simulink library "motohawk_control_primitives_motoshare_lib"  (Simulink 6.3)
undefined symbols (not defined in the file or in its folder): motohawk_vardec_config_group, motohawk_vardec_path, p, samp_time, SampleTime
libraries: MotoHawk_lib x76, motohawk_control_primitives_lib x30, simulink x9
(part 1 of 3)
settings Model: Creator=Blake Suhre  LastModifiedBy=Jason_Tartt  StrictBusMsg=None

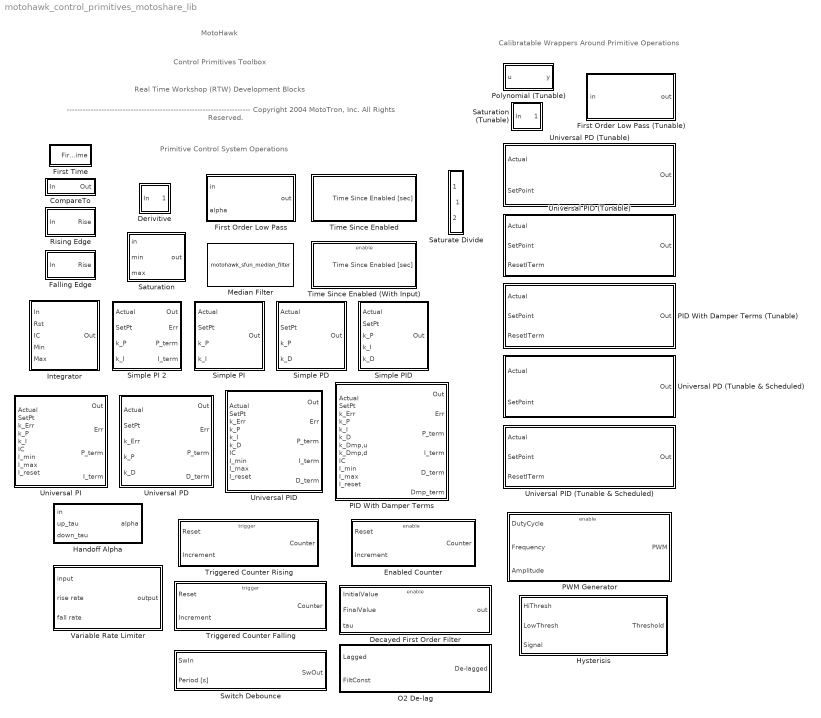
== system motohawk_control_primitives_motoshare_lib ==
  note: Calibratable Wrappers Around
      | Primitive Operations
  note: Primitive Control System Operations
  note: MotoHawk
  note: ---------------------------------------------------------------------
      | Copyright 2004 MotoTron, Inc.  All Rights Reserved.
  note: Real Time Workshop (RTW)
      | Development Blocks
  note: Control Primitives Toolbox
  CompareTo : Subsystem  mask(Equals){op===, val=1}
      mask prompts: op "Operator:"; val "Compare To:"
      mask help:
      | Check how input compares to 'n'.
      | Select an operation for comparison.
      | Any data type may be used for the value.  Real data type is based on input signal.
      mask init:
      | lbl = sprintf('in %s %d', op, double(val));
      | set_param([gcb '/RelOp'], 'Operator', op);
      mask StyleString: popup(==|~=|<|<=|>|>=),edit
      mask Display:
      | patch([0 0 1 1], 1.2*[0 0.075 0.075 0], [230/255 0/255 0/255])
      | patch([0 0 1 1], 1.2*[0.025 0.05 0.05 0.025], [150/255 0/255 0/255])
      | patch([0 0 1 1], 1.2*[0 0.025 0.025 0], [0/255 0/255 0/255])
      | 
      | disp(lbl);
  Decayed First Order Filter : Subsystem
      mask Type: Decayed First-Order Filter
      mask Description:
      | Discrete first-order low-pass filter that decays from the Initial Value to the Final Value when enabled.
      | 
      | The 'alpha' input is T/t.  So when alpha = 1, the block simply passes the input through to the output, and when alpha = 0, the block forever holds its last output value.
      mask Display:
      | patch([0 0 1 1], [0 0.075 0.075 0], [230/255 0/255 0/255])
      | patch([0 0 1 1], [0.025 0.05 0.05 0.025], [150/255 0/255 0/255])
      | patch([0 0 1 1], [0 0.025 0.025 0], [0/255 0/255 0/255])
      | 
      | disp('Decayed 1st-Order\nLow Pass');
  Derivitive : Subsystem  mask(Discrete Derivative){samp_time=SampleTime}
      mask prompts: samp_time "Sample Time"
      mask help:
      | Discrete-time derivitive.
      |
      | If 'Sample Time' is -1, then extra code and RAM will be generated to dynamically calculate dt.
      mask Display:
      | patch([0 0 1 1], [0 0.075 0.075 0], [230/255 0/255 0/255])
      | patch([0 0 1 1], [0.025 0.05 0.05 0.025], [150/255 0/255 0/255])
      | patch([0 0 1 1], [0 0.025 0.025 0], [0/255 0/255 0/255])
      | 
      | disp('\bf\itd/dt', 'texmode', 'on')
  Enabled Counter : Subsystem  TreatAsAtomicUnit=on
      mask Display:
      | patch([0 0 1 1], [0 0.075 0.075 0], [230/255 0/255 0/255])
      | patch([0 0 1 1], [0.025 0.05 0.05 0.025], [150/255 0/255 0/255])
      | patch([0 0 1 1], [0 0.025 0.025 0], [0/255 0/255 0/255])
      | 
      | disp(['ENABLED\nCOUNTER'])
  Falling Edge : Subsystem
      mask Display:
      | patch([0 0 1 1], [0 0.075 0.075 0], [230/255 0/255 0/255])
      | patch([0 0 1 1], [0.025 0.05 0.05 0.025], [150/255 0/255 0/255])
      | patch([0 0 1 1], [0 0.025 0.025 0], [0/255 0/255 0/255])
      | 
      | disp('Falling\nEdge');
  First Order Low Pass : Subsystem
      mask Type: First-Order Low-Pass Filter
      mask Description:
      | Discrete first-order low-pass filter.
      | 
      | The 'alpha' input is T/t.  So when alpha = 1, the block simply passes the input through to the output, and when alpha = 0, the block forever holds its last output value.
      mask Display:
      | patch([0 0 1 1], [0 0.075 0.075 0], [230/255 0/255 0/255])
      | patch([0 0 1 1], [0.025 0.05 0.05 0.025], [150/255 0/255 0/255])
      | patch([0 0 1 1], [0 0.025 0.025 0], [0/255 0/255 0/255])
      | 
      | disp('1st-Order\nLow Pass');
  First Order Low Pass (Tunable) : Subsystem  mask(First-Order Low-Pass Filter (Tunable)){nam='FiltConst', samp_time=-1, group=motohawk_vardec_path(gcb)}
      mask prompts: nam "Name"; samp_time "Sample Time"; group "MotoTune Group String"
      mask help:
      | Discrete first-order low-pass filter, with calibratable time-constant.
      |
      | If 'Sample Time' is -1, then extra code and RAM will be generated to dynamically calculate dt.
      mask Display:
      | patch([0 0 1 1], [0 0.075 0.075 0], [230/255 0/255 0/255])
      | patch([0 0 1 1], [0.025 0.05 0.05 0.025], [150/255 0/255 0/255])
      | patch([0 0 1 1], [0 0.025 0.025 0], [0/255 0/255 0/255])
      | 
      | disp('1st-Order\nLow Pass');
  First Time : Subsystem
      mask Display:
      | patch([0 0 1 1], [0 0.075 0.075 0], [230/255 0/255 0/255])
      | patch([0 0 1 1], [0.025 0.05 0.05 0.025], [150/255 0/255 0/255])
      | patch([0 0 1 1], [0 0.025 0.025 0], [0/255 0/255 0/255])
  Handoff Alpha : Subsystem  mask{samp_time=-1}
      mask prompts: samp_time "SampleTime"
      mask Display:
      | patch([0 0 1 1], [0 0.075 0.075 0], [230/255 0/255 0/255])
      | patch([0 0 1 1], [0.025 0.05 0.05 0.025], [150/255 0/255 0/255])
      | patch([0 0 1 1], [0 0.025 0.025 0], [0/255 0/255 0/255])
      | 
      | plot([.3 .4 .6 .8], [.3 .8 .8 .3]);
  Hysterisis : Subsystem
      mask Display:
      | patch([0 0 1 1], [0 0.075 0.075 0], [230/255 0/255 0/255])
      | patch([0 0 1 1], [0.025 0.05 0.05 0.025], [150/255 0/255 0/255])
      | patch([0 0 1 1], [0 0.025 0.025 0], [0/255 0/255 0/255])
      | 
      | disp('HYSTERISIS')
  Integrator : Subsystem  mask(Discrete Integrator){samp_time=samp_time}
      mask prompts: samp_time "Sample Time"
      mask help:
      | Resetable integrator with upper and lower windup limits.
      |
      | If 'Sample Time' is -1, then extra code and RAM will be generated to dynamically calculate dt.
      mask Display:
      | patch([0 0 1 1], 0.75*[0 0.075 0.075 0], [230/255 0/255 0/255])
      | patch([0 0 1 1], 0.75*[0.025 0.05 0.05 0.025], [150/255 0/255 0/255])
      | patch([0 0 1 1], 0.75*[0 0.025 0.025 0], [0/255 0/255 0/255])
      | 
      | disp('\fontsize{16}\bf\it\int dt', 'texmode', 'on')
  Median Filter : S-Function  FunctionName=motohawk_sfun_median_filter  Parameters=uint32(buffer_size)  mask(MotoHawk Median Filter){buffer_size=7}
      mask prompts: buffer_size "Buffer Size"
      mask help:
      | Maintains a buffer of 'Buffer Size' values, and outputs the median value stored in the buffer.
      |
      | ---------------------------------------------------------------------
      | Copyright 2004 MotoTron, Inc.  All Rights Reserved.
      mask init:
      | lbl = sprintf('Median Filter\nBuffer Size: %d', floor(double(buffer_size)));
      mask Display:
      | patch([0 0 1 1], [0 0.075 0.075 0], [230/255 0/255 0/255])
      | patch([0 0 1 1], [0.025 0.05 0.05 0.025], [150/255 0/255 0/255])
      | patch([0 0 1 1], [0 0.025 0.025 0], [0/255 0/255 0/255])
      | 
      | disp(lbl);
  O2 De-lag : Subsystem
      mask Display:
      | patch([0 0 1 1], [0 0.075 0.075 0], [230/255 0/255 0/255])
      | patch([0 0 1 1], [0.025 0.05 0.05 0.025], [150/255 0/255 0/255])
      | patch([0 0 1 1], [0 0.025 0.025 0], [0/255 0/255 0/255])
      | 
      | disp('First Order \nDe-Lag');
  PID With Damper Terms : Subsystem  Description=|  mask(PID with Damper Terms){samp_time=-1}
      | /* Name: ErrorGain Unit:mult ClassID:VAR StorageID:FLASH Access:RW4+RW3+NA2+NA1 TypeID:UINT4                   
      |    Gain:0.000000001 Min:0.000000000 Max:4.000000000 Format:10.9 UpdateID:REMOTE Help:"This gain is applied to "
      |    "the error term before it is used to calculate the P, I and D terms." VardecSig:6C */                       
      |                                                                                                                
      | /* Name: ITermLowerLim Unit:0 ClassID:VAR StorageID:FLASH Access:RW4+RW3+NA2+NA1 TypeID:SINT2 Gain:0.1         
      |    Min:-3276.8 Max:3276.7 Format:5.1 UpdateID:REMOTE Help:"Lower limit on the I-term value." VardecSig:6C */   
      |                                                                                                                
      | /* Name: ITermUpperLim ClassID:VAR StorageID:FLASH Access:RW4+RW3+NA2+NA1 TypeID:SINT2 Gain:0.1 Min:-3276.8    
      |    Max:3276.7 Format:5.1 UpdateID:REMOTE Help:"Upper limit on I-term value." VardecSig:6C */                   
      |                                                                                                                
      | /* Name: PIDOutLowerLim ClassID:VAR StorageID:FLASH Access:RW4+RW3+NA2+NA1 TypeID:SINT2 Gain:0.1               
      |    Min:-3276.8 Max:3276.7 Format:5.1 UpdateID:REMOTE Help:"Lower limit on PID output." VardecSig:6C */         
      |                                                                                                                
      | /* Name: PIDOutUpperLim ClassID:VAR StorageID:FLASH Access:RW4+RW3+NA2+NA1 TypeID:SINT2 Gain:0.1               
      |    Min:-3276.8 Max:3276.7 Format:3.1 UpdateID:REMOTE Help:"Upper limit on PID output." VardecSig:6C */         
      |                                                                                                                
      | /* Name: PIDError ClassID:VAR StorageID:RAM Access:RO4+RO3+NA2+NA1 TypeID:SINT2 Gain:1 Min:-32768.00           
      |    Max:32767.00 Format:4.2 UpdateID:BACKGND Help:"Current controller error input value." VardecSig:6C */       
      |                                                                                                                
      | /* Name: PTerm ClassID:VAR StorageID:RAM Access:RO4+RO3+NA2+NA1 TypeID:SINT2 Gain:1 Min:-32768.00              
      |    Max:32767.00 Format:4.2 UpdateID:BACKGND Help:"Current P-term value" VardecSig:6C */                        
      |                                                                                                                
      | /* Name: ITerm ClassID:VAR StorageID:RAM Access:RO4+RO3+NA2+NA1 TypeID:SINT2 Gain:1 Min:-32768.00              
      |    Max:32767.00 Format:4.2 UpdateID:BACKGND Help:"Current I-term value" VardecSig:6C */                        
      |                                                                                                                
      | /* Name: DTerm ClassID:VAR StorageID:RAM Access:RO4+RO3+NA2+NA1 TypeID:SINT2 Gain:1 Min:-32768.00              
      |    Max:32767.00 Format:4.2 UpdateID:BACKGND Help:"Current D-term value" VardecSig:6C */                        
      |                                                                                                                
      | /* Name: DamperTerm ClassID:VAR StorageID:RAM Access:RO4+RO3+NA2+NA1 TypeID:SINT2 Gain:1 Min:-32768.00         
      |    Max:32767.00 Format:4.2 UpdateID:BACKGND Help:"Current Damper-term value" VardecSig:6C */                   
      |                                                                                                                
      | /* Name: PIDOutput ClassID:VAR StorageID:FLASH Access:RW4+RW3+NA2+NA1 TypeID:SINT2 Gain:1 Min:-32768.00        
      |    Max:32767.00 Format:4.2 UpdateID:REMOTE Help:"PID current output." VardecSig:6C */
      mask prompts: samp_time "Sample Time"
      mask help:
      | Resettable PID controller with damper terms and limits on the I-term.
      |
      | If 'Sample Time' is -1, then extra code and RAM will be generated to dynamically calculate dt.
      mask Display:
      | patch([0 0 1 1], 0.5*[0 0.075 0.075 0], [230/255 0/255 0/255])
      | patch([0 0 1 1], 0.5*[0.025 0.05 0.05 0.025], [150/255 0/255 0/255])
      | patch([0 0 1 1], 0.5*[0 0.025 0.025 0], [0/255 0/255 0/255])
      | 
      | disp('\fontsize{16}\bf\itPIDD', 'texmode', 'on')
  PID With Damper Terms (Tunable) : Subsystem  mask(PID with Damper Terms (Tunable)){nam='Electronic Throttle Control', prefix='ETC_', samp_time=-1, units='', grp='Actuators | ETC'}
      mask prompts: nam "Name"; samp_time "Sample Time"; grp "MotoTune Group String"
      mask help:
      | This block wraps a 'PID With Damper Terms' block to provide calibrations and probes for most parameters.
      |
      | If 'Sample Time' is -1, then extra code and RAM will be generated to dynamically calculate dt.
      mask Display:
      | patch([0 0 1 1], [0 0.075 0.075 0], [230/255 0/255 0/255])
      | patch([0 0 1 1], [0.025 0.05 0.05 0.025], [150/255 0/255 0/255])
      | patch([0 0 1 1], [0 0.025 0.025 0], [0/255 0/255 0/255])
      | 
      | disp([nam '\n(PIDD)']);
  PWM Generator : Subsystem  TreatAsAtomicUnit=on
      mask Display:
      | patch([0 0 1 1], [0 0.075 0.075 0], [230/255 0/255 0/255])
      | patch([0 0 1 1], [0.025 0.05 0.05 0.025], [150/255 0/255 0/255])
      | patch([0 0 1 1], [0 0.025 0.025 0], [0/255 0/255 0/255])
      | 
      | disp('ENABLED\nPWM\nGENERATOR')
  Polynomial (Tunable) : Subsystem  mask(Polynomial (Tunable)){prefix='SamplePoly', numcoef=6, grp=motohawk_vardec_path(gcb)}
      mask prompts: numcoef "Number Of Coefficients"; grp "MotoTune Group String"
      mask help: Polynomial evaluation block with calibratable coefficients and centering/scaling parameters.
      mask Display:
      | patch([0 0 1 1], [0 0.075 0.075 0], [230/255 0/255 0/255])
      | patch([0 0 1 1], [0.025 0.05 0.05 0.025], [150/255 0/255 0/255])
      | patch([0 0 1 1], [0 0.025 0.025 0], [0/255 0/255 0/255])
      | 
      | disp(['P(u)\nO(P)'])
  Rising Edge : Subsystem
      mask Display:
      | patch([0 0 1 1], [0 0.075 0.075 0], [230/255 0/255 0/255])
      | patch([0 0 1 1], [0.025 0.05 0.05 0.025], [150/255 0/255 0/255])
      | patch([0 0 1 1], [0 0.025 0.025 0], [0/255 0/255 0/255])
      | 
      | disp('Rising\nEdge');
  Saturate Divide : Subsystem
      mask Display:
      | patch([0 0 1 1], [0 0.075 0.075 0], [230/255 0/255 0/255])
      | patch([0 0 1 1], [0.025 0.05 0.05 0.025], [150/255 0/255 0/255])
      | patch([0 0 1 1], [0 0.025 0.025 0], [0/255 0/255 0/255])
  Saturation : Subsystem  mask(Saturation){}
      mask help: Saturation block.
      mask Display:
      | patch([0 0 1 1], [0 0.075 0.075 0], [230/255 0/255 0/255])
      | patch([0 0 1 1], [0.025 0.05 0.05 0.025], [150/255 0/255 0/255])
      | patch([0 0 1 1], [0 0.025 0.025 0], [0/255 0/255 0/255])
      | 
      | plot([.2 .4 .6 .8], [.2 .2 .9 .9])
  Saturation (Tunable) : Subsystem  mask(Saturation (Tunable)){prefix='Saturation', units='', grp=motohawk_vardec_path(gcb)}
      mask prompts: grp "MotoTune Group String"
      mask help: Saturation block with calibratable min/max values.
      mask Display:
      | patch([0 0 1 1], [0 0.075 0.075 0], [230/255 0/255 0/255])
      | patch([0 0 1 1], [0.025 0.05 0.05 0.025], [150/255 0/255 0/255])
      | patch([0 0 1 1], [0 0.025 0.025 0], [0/255 0/255 0/255])
      | 
      | plot([0 .2 .8 1], [.1 .1 1 1])
  Simple PD : Subsystem  Description=|  mask(Universal PD){samp_time=-1}
      | /* Name: ErrorGain Unit:mult ClassID:VAR StorageID:FLASH Access:RW4+RW3+NA2+NA1 TypeID:UINT4                   
      |    Gain:0.000000001 Min:0.000000000 Max:4.000000000 Format:10.9 UpdateID:REMOTE Help:"This gain is applied to "
      |    "the error term before it is used to calculate the P, I and D terms." VardecSig:6C */                       
      |                                                                                                                
      | /* Name: ITermLowerLim Unit:0 ClassID:VAR StorageID:FLASH Access:RW4+RW3+NA2+NA1 TypeID:SINT2 Gain:0.1         
      |    Min:-3276.8 Max:3276.7 Format:5.1 UpdateID:REMOTE Help:"Lower limit on the I-term value." VardecSig:6C */   
      |                                                                                                                
      | /* Name: ITermUpperLim ClassID:VAR StorageID:FLASH Access:RW4+RW3+NA2+NA1 TypeID:SINT2 Gain:0.1 Min:-3276.8    
      |    Max:3276.7 Format:5.1 UpdateID:REMOTE Help:"Upper limit on I-term value." VardecSig:6C */                   
      |                                                                                                                
      | /* Name: PIDOutLowerLim ClassID:VAR StorageID:FLASH Access:RW4+RW3+NA2+NA1 TypeID:SINT2 Gain:0.1               
      |    Min:-3276.8 Max:3276.7 Format:5.1 UpdateID:REMOTE Help:"Lower limit on PID output." VardecSig:6C */         
      |                                                                                                                
      | /* Name: PIDOutUpperLim ClassID:VAR StorageID:FLASH Access:RW4+RW3+NA2+NA1 TypeID:SINT2 Gain:0.1               
      |    Min:-3276.8 Max:3276.7 Format:3.1 UpdateID:REMOTE Help:"Upper limit on PID output." VardecSig:6C */
      mask prompts: samp_time "Sample Time"
      mask help:
      | Resettable PD controller.
      |
      | If 'Sample Time' is -1, then extra code and RAM will be generated to dynamically calculate dt.
      mask Display:
      | patch([0 0 1 1], 0.75*[0 0.075 0.075 0], [230/255 0/255 0/255])
      | patch([0 0 1 1], 0.75*[0.025 0.05 0.05 0.025], [150/255 0/255 0/255])
      | patch([0 0 1 1], 0.75*[0 0.025 0.025 0], [0/255 0/255 0/255])
      | 
      | disp('\fontsize{16}\bf\itPD', 'texmode', 'on');
  Simple PI : Subsystem  Description=|  mask(Universal PID){samp_time=-1}
      | /* Name: ErrorGain Unit:mult ClassID:VAR StorageID:FLASH Access:RW4+RW3+NA2+NA1 TypeID:UINT4                   
      |    Gain:0.000000001 Min:0.000000000 Max:4.000000000 Format:10.9 UpdateID:REMOTE Help:"This gain is applied to "
      |    "the error term before it is used to calculate the P, I and D terms." VardecSig:6C */                       
      |                                                                                                                
      | /* Name: ITermLowerLim Unit:0 ClassID:VAR StorageID:FLASH Access:RW4+RW3+NA2+NA1 TypeID:SINT2 Gain:0.1         
      |    Min:-3276.8 Max:3276.7 Format:5.1 UpdateID:REMOTE Help:"Lower limit on the I-term value." VardecSig:6C */   
      |                                                                                                                
      | /* Name: ITermUpperLim ClassID:VAR StorageID:FLASH Access:RW4+RW3+NA2+NA1 TypeID:SINT2 Gain:0.1 Min:-3276.8    
      |    Max:3276.7 Format:5.1 UpdateID:REMOTE Help:"Upper limit on I-term value." VardecSig:6C */                   
      |                                                                                                                
      | /* Name: PIDOutLowerLim ClassID:VAR StorageID:FLASH Access:RW4+RW3+NA2+NA1 TypeID:SINT2 Gain:0.1               
      |    Min:-3276.8 Max:3276.7 Format:5.1 UpdateID:REMOTE Help:"Lower limit on PID output." VardecSig:6C */         
      |                                                                                                                
      | /* Name: PIDOutUpperLim ClassID:VAR StorageID:FLASH Access:RW4+RW3+NA2+NA1 TypeID:SINT2 Gain:0.1               
      |    Min:-3276.8 Max:3276.7 Format:3.1 UpdateID:REMOTE Help:"Upper limit on PID output." VardecSig:6C */
      mask prompts: samp_time "Sample Time"
      mask help:
      | Resettable PID controller with limits on the I-term.
      |
      | If 'Sample Time' is -1, then extra code and RAM will be generated to dynamically calculate dt.
      mask Display:
      | patch([0 0 1 1], 0.75*[0 0.075 0.075 0], [230/255 0/255 0/255])
      | patch([0 0 1 1], 0.75*[0.025 0.05 0.05 0.025], [150/255 0/255 0/255])
      | patch([0 0 1 1], 0.75*[0 0.025 0.025 0], [0/255 0/255 0/255])
      | 
      | disp('\fontsize{16}\bf\itPI', 'texmode', 'on');
  Simple PI 2 : Subsystem  Description=|  mask(Universal PID){samp_time=-1}
      | /* Name: ErrorGain Unit:mult ClassID:VAR StorageID:FLASH Access:RW4+RW3+NA2+NA1 TypeID:UINT4                   
      |    Gain:0.000000001 Min:0.000000000 Max:4.000000000 Format:10.9 UpdateID:REMOTE Help:"This gain is applied to "
      |    "the error term before it is used to calculate the P, I and D terms." VardecSig:6C */                       
      |                                                                                                                
      | /* Name: ITermLowerLim Unit:0 ClassID:VAR StorageID:FLASH Access:RW4+RW3+NA2+NA1 TypeID:SINT2 Gain:0.1         
      |    Min:-3276.8 Max:3276.7 Format:5.1 UpdateID:REMOTE Help:"Lower limit on the I-term value." VardecSig:6C */   
      |                                                                                                                
      | /* Name: ITermUpperLim ClassID:VAR StorageID:FLASH Access:RW4+RW3+NA2+NA1 TypeID:SINT2 Gain:0.1 Min:-3276.8    
      |    Max:3276.7 Format:5.1 UpdateID:REMOTE Help:"Upper limit on I-term value." VardecSig:6C */                   
      |                                                                                                                
      | /* Name: PIDOutLowerLim ClassID:VAR StorageID:FLASH Access:RW4+RW3+NA2+NA1 TypeID:SINT2 Gain:0.1               
      |    Min:-3276.8 Max:3276.7 Format:5.1 UpdateID:REMOTE Help:"Lower limit on PID output." VardecSig:6C */         
      |                                                                                                                
      | /* Name: PIDOutUpperLim ClassID:VAR StorageID:FLASH Access:RW4+RW3+NA2+NA1 TypeID:SINT2 Gain:0.1               
      |    Min:-3276.8 Max:3276.7 Format:3.1 UpdateID:REMOTE Help:"Upper limit on PID output." VardecSig:6C */
      mask prompts: samp_time "Sample Time"
      mask help:
      | Resettable PID controller with limits on the I-term.
      |
      | If 'Sample Time' is -1, then extra code and RAM will be generated to dynamically calculate dt.
      mask Display:
      | patch([0 0 1 1], 0.75*[0 0.075 0.075 0], [230/255 0/255 0/255])
      | patch([0 0 1 1], 0.75*[0.025 0.05 0.05 0.025], [150/255 0/255 0/255])
      | patch([0 0 1 1], 0.75*[0 0.025 0.025 0], [0/255 0/255 0/255])
      | 
      | disp('\fontsize{16}\bf\itPI', 'texmode', 'on');
  Simple PID : Subsystem  Description=|  mask(Universal PID){samp_time=-1}
      | /* Name: ErrorGain Unit:mult ClassID:VAR StorageID:FLASH Access:RW4+RW3+NA2+NA1 TypeID:UINT4                   
      |    Gain:0.000000001 Min:0.000000000 Max:4.000000000 Format:10.9 UpdateID:REMOTE Help:"This gain is applied to "
      |    "the error term before it is used to calculate the P, I and D terms." VardecSig:6C */                       
      |                                                                                                                
      | /* Name: ITermLowerLim Unit:0 ClassID:VAR StorageID:FLASH Access:RW4+RW3+NA2+NA1 TypeID:SINT2 Gain:0.1         
      |    Min:-3276.8 Max:3276.7 Format:5.1 UpdateID:REMOTE Help:"Lower limit on the I-term value." VardecSig:6C */   
      |                                                                                                                
      | /* Name: ITermUpperLim ClassID:VAR StorageID:FLASH Access:RW4+RW3+NA2+NA1 TypeID:SINT2 Gain:0.1 Min:-3276.8    
      |    Max:3276.7 Format:5.1 UpdateID:REMOTE Help:"Upper limit on I-term value." VardecSig:6C */                   
      |                                                                                                                
      | /* Name: PIDOutLowerLim ClassID:VAR StorageID:FLASH Access:RW4+RW3+NA2+NA1 TypeID:SINT2 Gain:0.1               
      |    Min:-3276.8 Max:3276.7 Format:5.1 UpdateID:REMOTE Help:"Lower limit on PID output." VardecSig:6C */         
      |                                                                                                                
      | /* Name: PIDOutUpperLim ClassID:VAR StorageID:FLASH Access:RW4+RW3+NA2+NA1 TypeID:SINT2 Gain:0.1               
      |    Min:-3276.8 Max:3276.7 Format:3.1 UpdateID:REMOTE Help:"Upper limit on PID output." VardecSig:6C */
      mask prompts: samp_time "Sample Time"
      mask help:
      | Resettable PID controller with limits on the I-term.
      |
      | If 'Sample Time' is -1, then extra code and RAM will be generated to dynamically calculate dt.
      mask Display:
      | patch([0 0 1 1], 0.75*[0 0.075 0.075 0], [230/255 0/255 0/255])
      | patch([0 0 1 1], 0.75*[0.025 0.05 0.05 0.025], [150/255 0/255 0/255])
      | patch([0 0 1 1], 0.75*[0 0.025 0.025 0], [0/255 0/255 0/255])
      | 
      | disp('\fontsize{16}\bf\itPID', 'texmode', 'on');
  Switch Debounce : Subsystem
      mask Display:
      | patch([0 0 1 1], [0 0.075 0.075 0], [230/255 0/255 0/255])
      | patch([0 0 1 1], [0.025 0.05 0.05 0.025], [150/255 0/255 0/255])
      | patch([0 0 1 1], [0 0.025 0.025 0], [0/255 0/255 0/255])
      | 
      | disp('SWITCH DEBOUNCE');
  Time Since Enabled : Subsystem  mask(Time Since Enabled){samp_time=-1}
      mask prompts: samp_time "Sample Time"
      mask help:
      | Outputs the amount of time that has elapsed since the enable input has gone high.
      |
      | Holds its value when the enable input goes low, but resets again when it goes high.
      |
      | If 'Sample Time' is -1, then extra code and RAM will be generated to dynamically calculate dt.
      mask Display:
      | patch([0 0 1 1], [0 0.075 0.075 0], [230/255 0/255 0/255])
      | patch([0 0 1 1], [0.025 0.05 0.05 0.025], [150/255 0/255 0/255])
      | patch([0 0 1 1], [0 0.025 0.025 0], [0/255 0/255 0/255])
      | 
      | disp('Time Since Enabled\n[sec]');
  Time Since Enabled (With Input) : Subsystem  mask(Time Since Enabled){samp_time=-1, init=0}
      mask prompts: samp_time "Sample Time"; init "Output When Disabled"
      mask help:
      | Outputs the amount of time that has elapsed since the enable input has gone high.
      |
      | Holds its value when the enable input goes low, but resets again when it goes high.
      |
      | If 'Sample Time' is -1, then extra code and RAM will be generated to dynamically calculate dt.
      mask Display:
      | patch([0 0 1 1], [0 0.075 0.075 0], [230/255 0/255 0/255])
      | patch([0 0 1 1], [0.025 0.05 0.05 0.025], [150/255 0/255 0/255])
      | patch([0 0 1 1], [0 0.025 0.025 0], [0/255 0/255 0/255])
      | 
      | disp('Time Since Enabled\n[sec]');
  Triggered Counter Falling : Subsystem  TreatAsAtomicUnit=on
      mask Type: MotoHawk Engine Physics:  No Adapt Counter
      mask Description:
      | ---------------------------------------------------------------------
      | Copyright 2004 MotoTron Corp.  All Rights Reserved.
      mask Display:
      | patch([0 0 1 1], [0 0.075 0.075 0], [230/255 0/255 0/255])
      | patch([0 0 1 1], [0.025 0.05 0.05 0.025], [150/255 0/255 0/255])
      | patch([0 0 1 1], [0 0.025 0.025 0], [0/255 0/255 0/255])
      | 
      | disp(['TRIGGERED\nCOUNTER\n(Falling Edge)'])
  Triggered Counter Rising : Subsystem  TreatAsAtomicUnit=on
      mask Type: MotoHawk Engine Physics:  No Adapt Counter
      mask Description:
      | ---------------------------------------------------------------------
      | Copyright 2004 MotoTron Corp.  All Rights Reserved.
      mask Display:
      | patch([0 0 1 1], [0 0.075 0.075 0], [230/255 0/255 0/255])
      | patch([0 0 1 1], [0.025 0.05 0.05 0.025], [150/255 0/255 0/255])
      | patch([0 0 1 1], [0 0.025 0.025 0], [0/255 0/255 0/255])
      | 
      | disp(['TRIGGERED\nCOUNTER\n(Rising Edge)'])
  Universal PD : Subsystem  Description=|  mask(Universal PD){samp_time=-1}
      | /* Name: ErrorGain Unit:mult ClassID:VAR StorageID:FLASH Access:RW4+RW3+NA2+NA1 TypeID:UINT4                   
      |    Gain:0.000000001 Min:0.000000000 Max:4.000000000 Format:10.9 UpdateID:REMOTE Help:"This gain is applied to "
      |    "the error term before it is used to calculate the P, I and D terms." VardecSig:6C */                       
      |                                                                                                                
      | /* Name: ITermLowerLim Unit:0 ClassID:VAR StorageID:FLASH Access:RW4+RW3+NA2+NA1 TypeID:SINT2 Gain:0.1         
      |    Min:-3276.8 Max:3276.7 Format:5.1 UpdateID:REMOTE Help:"Lower limit on the I-term value." VardecSig:6C */   
      |                                                                                                                
      | /* Name: ITermUpperLim ClassID:VAR StorageID:FLASH Access:RW4+RW3+NA2+NA1 TypeID:SINT2 Gain:0.1 Min:-3276.8    
      |    Max:3276.7 Format:5.1 UpdateID:REMOTE Help:"Upper limit on I-term value." VardecSig:6C */                   
      |                                                                                                                
      | /* Name: PIDOutLowerLim ClassID:VAR StorageID:FLASH Access:RW4+RW3+NA2+NA1 TypeID:SINT2 Gain:0.1               
      |    Min:-3276.8 Max:3276.7 Format:5.1 UpdateID:REMOTE Help:"Lower limit on PID output." VardecSig:6C */         
      |                                                                                                                
      | /* Name: PIDOutUpperLim ClassID:VAR StorageID:FLASH Access:RW4+RW3+NA2+NA1 TypeID:SINT2 Gain:0.1               
      |    Min:-3276.8 Max:3276.7 Format:3.1 UpdateID:REMOTE Help:"Upper limit on PID output." VardecSig:6C */
      mask prompts: samp_time "Sample Time"
      mask help:
      | Resettable PD controller.
      |
      | If 'Sample Time' is -1, then extra code and RAM will be generated to dynamically calculate dt.
      mask Display:
      | patch([0 0 1 1], 0.5*[0 0.075 0.075 0], [230/255 0/255 0/255])
      | patch([0 0 1 1], 0.5*[0.025 0.05 0.05 0.025], [150/255 0/255 0/255])
      | patch([0 0 1 1], 0.5*[0 0.025 0.025 0], [0/255 0/255 0/255])
      | 
      | disp('\fontsize{16}\bf\itPD', 'texmode', 'on');
  Universal PD (Tunable & Scheduled) : Subsystem  mask(Universal PD (Tunable)){nam='Idle Spark PD', prefix='IdleSpark_', samp_time=SampleTime, units='degCA', tblsize=10, group='Engine Control | Run | Idle Control'}
      mask prompts: nam "Name"; samp_time "Sample Time"; tblsize "Gain Schedule Table Size"; group "MotoTune Group String"
      mask help:
      | This block wraps a 'Universal PD' block to provide gain scheduling and calibrations and probes for most parameters.
      |
      | If 'Sample Time' is -1, then extra code and RAM will be generated to dynamically calculate dt.
      mask init:
      | grp = [group ' | ' nam];
      mask Display:
      | patch([0 0 1 1], [0 0.075 0.075 0], [230/255 0/255 0/255])
      | patch([0 0 1 1], [0.025 0.05 0.05 0.025], [150/255 0/255 0/255])
      | patch([0 0 1 1], [0 0.025 0.025 0], [0/255 0/255 0/255])
      | 
      | disp([nam '\n(PD w/ Gain Schedules)']);
  Universal PD (Tunable) : Subsystem  mask(Universal PD (Tunable)){nam='Idle Spark Control', prefix='IdleSpark_', samp_time=SampleTime, units='', group='Engine Control | Run | Idle Control'}
      mask prompts: nam "Name"; samp_time "Sample Time"; group "MotoTune Group String"
      mask help:
      | This block wraps a 'Universal PD' block to provide calibrations and probes for most parameters.
      |
      | If 'Sample Time' is -1, then extra code and RAM will be generated to dynamically calculate dt.
      mask init:
      | grp = [group ' | ' nam];
      mask Display:
      | patch([0 0 1 1], [0 0.075 0.075 0], [230/255 0/255 0/255])
      | patch([0 0 1 1], [0.025 0.05 0.05 0.025], [150/255 0/255 0/255])
      | patch([0 0 1 1], [0 0.025 0.025 0], [0/255 0/255 0/255])
      | 
      | disp([nam '\n(PD)']);
  Universal PI : Subsystem  Description=|  mask(Universal PID){samp_time=-1}
      | /* Name: ErrorGain Unit:mult ClassID:VAR StorageID:FLASH Access:RW4+RW3+NA2+NA1 TypeID:UINT4                   
      |    Gain:0.000000001 Min:0.000000000 Max:4.000000000 Format:10.9 UpdateID:REMOTE Help:"This gain is applied to "
      |    "the error term before it is used to calculate the P, I and D terms." VardecSig:6C */                       
      |                                                                                                                
      | /* Name: ITermLowerLim Unit:0 ClassID:VAR StorageID:FLASH Access:RW4+RW3+NA2+NA1 TypeID:SINT2 Gain:0.1         
      |    Min:-3276.8 Max:3276.7 Format:5.1 UpdateID:REMOTE Help:"Lower limit on the I-term value." VardecSig:6C */   
      |                                                                                                                
      | /* Name: ITermUpperLim ClassID:VAR StorageID:FLASH Access:RW4+RW3+NA2+NA1 TypeID:SINT2 Gain:0.1 Min:-3276.8    
      |    Max:3276.7 Format:5.1 UpdateID:REMOTE Help:"Upper limit on I-term value." VardecSig:6C */                   
      |                                                                                                                
      | /* Name: PIDOutLowerLim ClassID:VAR StorageID:FLASH Access:RW4+RW3+NA2+NA1 TypeID:SINT2 Gain:0.1               
      |    Min:-3276.8 Max:3276.7 Format:5.1 UpdateID:REMOTE Help:"Lower limit on PID output." VardecSig:6C */         
      |                                                                                                                
      | /* Name: PIDOutUpperLim ClassID:VAR StorageID:FLASH Access:RW4+RW3+NA2+NA1 TypeID:SINT2 Gain:0.1               
      |    Min:-3276.8 Max:3276.7 Format:3.1 UpdateID:REMOTE Help:"Upper limit on PID output." VardecSig:6C */
      mask prompts: samp_time "Sample Time"
      mask help:
      | Resettable PID controller with limits on the I-term.
      |
      | If 'Sample Time' is -1, then extra code and RAM will be generated to dynamically calculate dt.
      mask Display:
      | patch([0 0 1 1], 0.5*[0 0.075 0.075 0], [230/255 0/255 0/255])
      | patch([0 0 1 1], 0.5*[0.025 0.05 0.05 0.025], [150/255 0/255 0/255])
      | patch([0 0 1 1], 0.5*[0 0.025 0.025 0], [0/255 0/255 0/255])
      | 
      | disp('\fontsize{16}\bf\itPI', 'texmode', 'on');
  Universal PID : Subsystem  Description=|  mask(Universal PID){samp_time=-1}
      | /* Name: ErrorGain Unit:mult ClassID:VAR StorageID:FLASH Access:RW4+RW3+NA2+NA1 TypeID:UINT4                   
      |    Gain:0.000000001 Min:0.000000000 Max:4.000000000 Format:10.9 UpdateID:REMOTE Help:"This gain is applied to "
      |    "the error term before it is used to calculate the P, I and D terms." VardecSig:6C */                       
      |                                                                                                                
      | /* Name: ITermLowerLim Unit:0 ClassID:VAR StorageID:FLASH Access:RW4+RW3+NA2+NA1 TypeID:SINT2 Gain:0.1         
      |    Min:-3276.8 Max:3276.7 Format:5.1 UpdateID:REMOTE Help:"Lower limit on the I-term value." VardecSig:6C */   
      |                                                                                                                
      | /* Name: ITermUpperLim ClassID:VAR StorageID:FLASH Access:RW4+RW3+NA2+NA1 TypeID:SINT2 Gain:0.1 Min:-3276.8    
      |    Max:3276.7 Format:5.1 UpdateID:REMOTE Help:"Upper limit on I-term value." VardecSig:6C */                   
      |                                                                                                                
      | /* Name: PIDOutLowerLim ClassID:VAR StorageID:FLASH Access:RW4+RW3+NA2+NA1 TypeID:SINT2 Gain:0.1               
      |    Min:-3276.8 Max:3276.7 Format:5.1 UpdateID:REMOTE Help:"Lower limit on PID output." VardecSig:6C */         
      |                                                                                                                
      | /* Name: PIDOutUpperLim ClassID:VAR StorageID:FLASH Access:RW4+RW3+NA2+NA1 TypeID:SINT2 Gain:0.1               
      |    Min:-3276.8 Max:3276.7 Format:3.1 UpdateID:REMOTE Help:"Upper limit on PID output." VardecSig:6C */
      mask prompts: samp_time "Sample Time"
      mask help:
      | Resettable PID controller with limits on the I-term.
      |
      | If 'Sample Time' is -1, then extra code and RAM will be generated to dynamically calculate dt.
      mask Display:
      | patch([0 0 1 1], 0.5*[0 0.075 0.075 0], [230/255 0/255 0/255])
      | patch([0 0 1 1], 0.5*[0.025 0.05 0.05 0.025], [150/255 0/255 0/255])
      | patch([0 0 1 1], 0.5*[0 0.025 0.025 0], [0/255 0/255 0/255])
      | 
      | disp('\fontsize{16}\bf\itPID', 'texmode', 'on');
  Universal PID (Tunable & Scheduled) : Subsystem  mask(Universal PID (Tunable)){nam='Idle Air PID', prefix='IdleAir_', samp_time=SampleTime, units='%', tblsize=10, group='Engine Control | Run | Idle Control'}
      mask prompts: nam "Name"; samp_time "Sample Time"; tblsize "Gain Schedule Table Size"; group "MotoTune Group String"
      mask help:
      | This block wraps a 'Universal PID' block to provide gain scheduling and calibrations and probes for most parameters.
      |
      | If 'Sample Time' is -1, then extra code and RAM will be generated to dynamically calculate dt.
      mask init:
      | grp = [group ' | ' nam];
      mask Display:
      | patch([0 0 1 1], [0 0.075 0.075 0], [230/255 0/255 0/255])
      | patch([0 0 1 1], [0.025 0.05 0.05 0.025], [150/255 0/255 0/255])
      | patch([0 0 1 1], [0 0.025 0.025 0], [0/255 0/255 0/255])
      | 
      | disp([nam '\n(PID w/ Gain Schedules)']);
  Universal PID (Tunable) : Subsystem  mask(Universal PID (Tunable)){nam='Idle Air Control', prefix='IdleAir_', samp_time=SampleTime, units='', group='Engine Control | Run | Idle Control'}
      mask prompts: nam "Name"; samp_time "Sample Time"; group "MotoTune Group String"
      mask help:
      | This block wraps a 'Universal PID' block to provide calibrations and probes for most parameters.
      |
      | If 'Sample Time' is -1, then extra code and RAM will be generated to dynamically calculate dt.
      mask init:
      | grp = [group ' | ' nam];
      mask Display:
      | patch([0 0 1 1], [0 0.075 0.075 0], [230/255 0/255 0/255])
      | patch([0 0 1 1], [0.025 0.05 0.05 0.025], [150/255 0/255 0/255])
      | patch([0 0 1 1], [0 0.025 0.025 0], [0/255 0/255 0/255])
      | 
      | disp([nam '\n(PID)']);
  Variable Rate Limiter : Subsystem  mask(Variable Rate Limiter){}
      mask help: Variable Rate Limiter Block
      mask Display:
      | patch([0 0 1 1], [0 0.075 0.075 0], [230/255 0/255 0/255])
      | patch([0 0 1 1], [0.025 0.05 0.05 0.025], [150/255 0/255 0/255])
      | patch([0 0 1 1], [0 0.025 0.025 0], [0/255 0/255 0/255])
      | 
      | disp(['RATE \nLIMITER']);

== system motohawk_control_primitives_motoshare_lib/CompareTo ==
  note: Check how input compares to 'val'
  In : Inport
  Constant : Constant  Value=val
  RelOp : RelationalOperator  Operator===  ZeroCross=off  InputSameDT=on
  Out : Outport
  wires:
  Constant/1 -> RelOp/2
  RelOp/1 -> Out/1
  In/1 -> RelOp/1

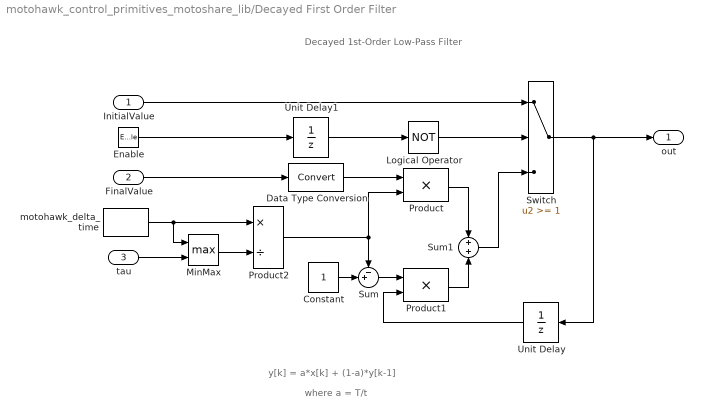
== system motohawk_control_primitives_motoshare_lib/Decayed First Order Filter ==
  note: where a = T/t
  note: Decayed 1st-Order Low-Pass Filter
  note: y[k] = a*x[k] + (1-a)*y[k-1]
  InitialValue : Inport
  FinalValue : Inport  Port=2
  tau : Inport  Port=3
  Enable : EnablePort  StatesWhenEnabling=reset  ShowOutputPort=on
  Constant : Constant
  Data Type Conversion : DataTypeConversion  SaturateOnIntegerOverflow=on  RndMeth=Zero
  Logical Operator : Logic  Operator=NOT  AllPortsSameDT=off
  MinMax : MinMax  Function=max  Inputs=2  SaturateOnIntegerOverflow=on  InputSameDT=on
  Product : Product  SaturateOnIntegerOverflow=on  InputSameDT=on
  Product1 : Product  SaturateOnIntegerOverflow=on  InputSameDT=on
  Product2 : Product  Inputs=*/  SaturateOnIntegerOverflow=on  InputSameDT=on
  Sum : Sum  Inputs=-+|  SaturateOnIntegerOverflow=on
  Sum1 : Sum  SaturateOnIntegerOverflow=on
  Switch : Switch  Threshold=1  SaturateOnIntegerOverflow=on
  Unit Delay : UnitDelay  Orientation=left  SampleTime=-1
  Unit Delay1 : UnitDelay  SampleTime=-1
  motohawk_delta_time : MotoHawk_lib/Extra Development Blocks/motohawk_delta_time  samp_time=-1  init_val=0
  out : Outport
  wires:
  Product2/1 -> Sum/1, Product/2
  Unit Delay1/1 -> Logical Operator/1
  Logical Operator/1 -> Switch/2
  InitialValue/1 -> Switch/1
  Enable/1 -> Unit Delay1/1
  Switch/1 -> Unit Delay/1, out/1
  Sum1/1 -> Switch/3
  Data Type Conversion/1 -> Product/1
  Unit Delay/1 -> Product1/2
  Sum/1 -> Product1/1
  Product1/1 -> Sum1/2
  Product/1 -> Sum1/1
  FinalValue/1 -> Data Type Conversion/1
  Constant/1 -> Sum/2
  motohawk_delta_time/1 -> Product2/1, MinMax/1
  MinMax/1 -> Product2/2
  tau/1 -> MinMax/2

== system motohawk_control_primitives_motoshare_lib/Derivitive ==
  note: Discrete Derivative
  In : Inport
  Product : Product  Inputs=*/  SaturateOnIntegerOverflow=on  InputSameDT=on
  Sum2 : Sum  Inputs=-+|  SaturateOnIntegerOverflow=on
  Unit Delay : UnitDelay  SampleTime=-1
  motohawk_delta_time : MotoHawk_lib/Extra Development Blocks/motohawk_delta_time  samp_time=samp_time  init_val=inf
  Out : Outport
  wires:
  Product/1 -> Out/1
  motohawk_delta_time/1 -> Product/2
  Sum2/1 -> Product/1
  In/1 -> Sum2/2, Unit Delay/1
  Unit Delay/1 -> Sum2/1

== system motohawk_control_primitives_motoshare_lib/Enabled Counter ==
  note: Enabled Counter
  Reset : Inport
  Increment : Inport  Port=2
  Enable : EnablePort
  Constant : Constant  Value=0
  Sum : Sum  Orientation=up  SaturateOnIntegerOverflow=on  InputSameDT=on
  Switch : Switch  Threshold=0.5  SaturateOnIntegerOverflow=on  InputSameDT=on
  Unit Delay2 : UnitDelay  SampleTime=-1
  Counter : Outport
  wires:
  Unit Delay2/1 -> Counter/1, Sum/2
  Switch/1 -> Unit Delay2/1
  Reset/1 -> Switch/2
  Constant/1 -> Switch/1
  Sum/1 -> Switch/3
  Increment/1 -> Sum/1

== system motohawk_control_primitives_motoshare_lib/Falling Edge ==
  note: Detect Falling Edge of Signal
      | using Discrete Unit Delay
  In : Inport
  Data Type Conversion : DataTypeConversion  OutDataTypeMode=boolean  SaturateOnIntegerOverflow=on  RndMeth=Zero
  Logical Operator : Logic
  Logical Operator2 : Logic  Operator=NOT
  Unit Delay : UnitDelay  SampleTime=-1
  Rise : Outport
  wires:
  Data Type Conversion/1 -> Logical Operator2/1, Unit Delay/1
  Logical Operator2/1 -> Logical Operator/1
  In/1 -> Data Type Conversion/1
  Logical Operator/1 -> Rise/1
  Unit Delay/1 -> Logical Operator/2

== system motohawk_control_primitives_motoshare_lib/First Order Low Pass ==
  note: where a = t/T
  note: 1st-Order Low-Pass Filter
  note: y[k] = a*x[k] + (1-a)*y[k-1]
  in : Inport
  alpha : Inport  Port=2
  Constant : Constant
  Data Type Conversion : DataTypeConversion  SaturateOnIntegerOverflow=on  RndMeth=Zero
  Product : Product  SaturateOnIntegerOverflow=on  InputSameDT=on
  Product1 : Product  SaturateOnIntegerOverflow=on  InputSameDT=on
  Sum : Sum  Inputs=-+|  SaturateOnIntegerOverflow=on
  Sum1 : Sum  SaturateOnIntegerOverflow=on
  Unit Delay : UnitDelay  Orientation=left  SampleTime=-1
  out : Outport
  wires:
  Data Type Conversion/1 -> Product/1
  Sum1/1 -> out/1, Unit Delay/1
  Unit Delay/1 -> Product1/2
  Sum/1 -> Product1/1
  Product1/1 -> Sum1/2
  Product/1 -> Sum1/1
  in/1 -> Data Type Conversion/1
  Constant/1 -> Sum/2
  alpha/1 -> Product/2, Sum/1

== system motohawk_control_primitives_motoshare_lib/First Order Low Pass (Tunable) ==
  note: Tunable 1st-Order Low-Pass Filter
  in : Inport
  First Order Low Pass : motohawk_control_primitives_lib/First Order Low Pass
  MinMax : MinMax  Function=max  Inputs=2  SaturateOnIntegerOverflow=on  InputSameDT=on
  Product : Product  Inputs=*/  SaturateOnIntegerOverflow=on  InputSameDT=on
  motohawk_calibration : MotoHawk_lib/Calibration & Probing Blocks/motohawk_calibration  nam=nam  val=.005  storage=Calibration  show_more=on  name_source=Use Parameter  data_type=Inherit from 'Default Value'  read_level=1  write_level=1  ovr_cals=on  view_as=Number  enum_struct={'Disabled', 'Enabled'}  vector_style=Wide Row  use_help_units=on  help='Filter time constant'  units='sec'  use_header_enum=off  row_header_enum={}  col_header_enum={}  use_min_max=off  min_val=-inf  max_val=inf  use_precision=off  precision=''  gain=1  offset=0  exp=1  use_mototune_group=on  mototune_group=group %% motohawk_vardec_config_group(group)
  motohawk_delta_time : MotoHawk_lib/Extra Development Blocks/motohawk_delta_time  samp_time=samp_time  init_val=0
  out : Outport
  wires:
  motohawk_calibration/1 -> MinMax/2
  MinMax/1 -> Product/2
  Product/1 -> First Order Low Pass/2
  motohawk_delta_time/1 -> MinMax/1, Product/1
  in/1 -> First Order Low Pass/1
  First Order Low Pass/1 -> out/1

== system motohawk_control_primitives_motoshare_lib/First Time ==
  False After First Sample : Constant  Value=false
  Initial Condition is True : UnitDelay  X0=true  SampleTime=-1
  First Time : Outport
  wires:
  Initial Condition is True/1 -> First Time/1
  False After First Sample/1 -> Initial Condition is True/1

== system motohawk_control_primitives_motoshare_lib/Handoff Alpha ==
  note: Prevent divide by zero
  note: Convert a boolean input signal
      | to a more slowly ramping 'alpha' from 0 to 1
  in : Inport
  up_tau : Inport  Port=2
  down_tau : Inport  Port=3
  Constant : Constant  Value=0
  Constant1 : Constant
  Multiport Switch : MultiPortSwitch  Inputs=2  zeroidx=on  SaturateOnIntegerOverflow=on  InputSameDT=on
  Product : Product  Inputs=*/  SaturateOnIntegerOverflow=on  InputSameDT=on
  Product1 : Product  Inputs=*/  SaturateOnIntegerOverflow=on  InputSameDT=on
  Ramp Down : Gain  Gain=-1  SaturateOnIntegerOverflow=on
  Saturation : motohawk_control_primitives_lib/Saturation
  Signal Specification : SignalSpecification  DataType=boolean
  Sum : Sum  Inputs=|++  SaturateOnIntegerOverflow=on  InputSameDT=on
  Switch : Switch  Criteria=u2 > Threshold  SaturateOnIntegerOverflow=on  InputSameDT=on
  Switch1 : Switch  Criteria=u2 > Threshold  SaturateOnIntegerOverflow=on  InputSameDT=on
  motohawk_delta_time : MotoHawk_lib/Extra Development Blocks/motohawk_delta_time  samp_time=samp_time  init_val=0
  state : UnitDelay  Orientation=left  SampleTime=-1
  alpha : Outport
  wires:
  up_tau/1 -> Switch1/1, Switch1/2
  Switch1/1 -> Product1/2
  down_tau/1 -> Switch/1, Switch/2
  Switch/1 -> Product/2
  Signal Specification/1 -> Multiport Switch/1
  Ramp Down/1 -> Multiport Switch/2
  Saturation/1 -> alpha/1, state/1
  Constant1/1 -> Saturation/3
  Constant/1 -> Saturation/2
  state/1 -> Sum/2
  Sum/1 -> Saturation/1
  Multiport Switch/1 -> Sum/1
  Product1/1 -> Multiport Switch/3
  Product/1 -> Ramp Down/1
  in/1 -> Signal Specification/1
  motohawk_delta_time/1 -> Switch1/3, Product1/1, Switch/3, Product/1

== system motohawk_control_primitives_motoshare_lib/Hysterisis ==
  HiThresh : Inport
  LowThresh : Inport  Port=2
  Signal : Inport  Port=3
  Hysteresis : Subsystem
  LT : RelationalOperator  ZeroCross=off  InputSameDT=on
  LT1 : RelationalOperator  Operator=<=  ZeroCross=off  InputSameDT=on
  Logical Operator : Logic  Operator=NOT
  Switch2 : Switch  Threshold=1  ZeroCross=off  InputSameDT=on
  Threshold : Outport
  wires:
  LT/1 -> Hysteresis/1(Hi)  "AboveHiTarget"
  LT1/1 -> Hysteresis/2(Lo)  "BelowLoTarget"
  Hysteresis/1("Out (Lo=0, Hi=1)") -> Logical Operator/1
  Logical Operator/1 -> Switch2/2
  HiThresh/1 -> Switch2/1, LT/2
  Switch2/1 -> Threshold/1
  LowThresh/1 -> Switch2/3, LT1/2
  Signal/1 -> LT/1, LT1/1

== system motohawk_control_primitives_motoshare_lib/Integrator ==
  note: Discrete Integrator,
      | with output and state saturation.
  In : Inport  Orientation=left
  Rst : Inport  Port=2
  IC : Inport  Port=3
  Min : Inport  Orientation=left  Port=4
  Max : Inport  Orientation=left  Port=5
  Data Type Conversion : DataTypeConversion  OutDataTypeMode=boolean  RndMeth=Zero
  Product : Product  Orientation=left  SaturateOnIntegerOverflow=on  InputSameDT=on
  Saturation : motohawk_control_primitives_lib/Saturation  Orientation=left
  Sum : Sum  Orientation=left  Inputs=++|  SaturateOnIntegerOverflow=on  InputSameDT=on
  Switch1 : Switch  Threshold=1  ZeroCross=off  SaturateOnIntegerOverflow=on  InputSameDT=on
  Unit Delay : UnitDelay  Orientation=left  SampleTime=-1
  motohawk_delta_time : MotoHawk_lib/Extra Development Blocks/motohawk_delta_time  Orientation=left  samp_time=samp_time  init_val=0
  Out : Outport
  wires:
  Saturation/1 -> Unit Delay/1
  Sum/1 -> Saturation/1
  Switch1/1 -> Sum/1, Out/1
  motohawk_delta_time/1 -> Product/2
  In/1 -> Product/1
  Product/1 -> Sum/2
  Unit Delay/1 -> Switch1/3
  Rst/1 -> Data Type Conversion/1
  Data Type Conversion/1 -> Switch1/2
  Min/1 -> Saturation/2
  Max/1 -> Saturation/3
  IC/1 -> Switch1/1

== system motohawk_control_primitives_motoshare_lib/O2 De-lag ==
  Lagged : Inport
  FiltConst : Inport  Port=2
  Constant : Constant
  MinMax : MinMax  Function=max  Inputs=2  SaturateOnIntegerOverflow=on  InputSameDT=on
  Product : Product  RndMeth=Zero
  Product1 : Product  RndMeth=Zero
  Product2 : Product  Inputs=*/  SaturateOnIntegerOverflow=on  InputSameDT=on
  Sum : Sum  Inputs=|+-
  Sum1 : Sum  Inputs=+|+
  Unit Delay : UnitDelay  SampleTime=-1
  motohawk_delta_time : MotoHawk_lib/Extra Development Blocks/motohawk_delta_time  samp_time=-1  init_val=0
  De-lagged : Outport
  wires:
  Sum1/1 -> De-lagged/1
  Product1/1 -> Sum1/1
  Product/1 -> Sum1/2
  Sum/1 -> Product1/2
  Unit Delay/1 -> Product1/1
  Constant/1 -> Sum/1
  Lagged/1 -> Unit Delay/1, Product/2
  MinMax/1 -> Product2/2
  motohawk_delta_time/1 -> MinMax/1, Product2/1
  Product2/1 -> Product/1, Sum/2
  FiltConst/1 -> MinMax/2
